simulink model "AOO_state"  (R2020a)
settings: Solver=FixedStepAuto  StartTime=0.0  StopTime=10.0  FixedStep=1e-3  RelTol=1e-3  EnableMultiTasking=on
undefined symbols (not defined in the file or in its folder): A1, D0, D1, D2, PTB3, PTB9, PTC16, PTC17
libraries: frdmk64flib x4
settings Model: ExtModeTrigDuration=5  Creator=John Sarga  LastModifiedBy=John Sarga
settings OptimizationCC: EnhancedBackFolding=on  PassReuseOutputArgsAs=Individual arguments  ZeroExternalMemoryAtStartup=off  ZeroInternalMemoryAtStartup=off  MaxStackSize=64  OptimizeBlockOrder=speed  DifferentSizesBufferReuse=on  OptimizationCustomize=off  EfficientTunableParamExpr=on
settings DebuggingCC: ParameterTunabilityLossMsg=error
settings HardwareCC: ProdBitPerPointer=32  ProdBitPerSizeT=32  ProdBitPerPtrDiffT=32  ProdLargestAtomicInteger=Long  ProdLargestAtomicFloat=Double  ProdWordSize=32  ProdHWDeviceType=ARM Compatible->ARM Cortex
settings SFSimCC: MATLABDynamicMemAlloc=off
settings RTWCC: SystemTargetFile=ert.tlc  HardwareBoard=NXP FRDM-K64F  TemplateMakefile=ert_default_tmf  Toolchain=GNU Tools for ARM Embedded Processors
settings CodeAppCC: ForceParamTrailComments=on  IgnoreCustomStorageClasses=off  OperatorAnnotations=on  SimulinkDataObjDesc=on  SFDataObjDesc=on  InsertBlockDesc=on

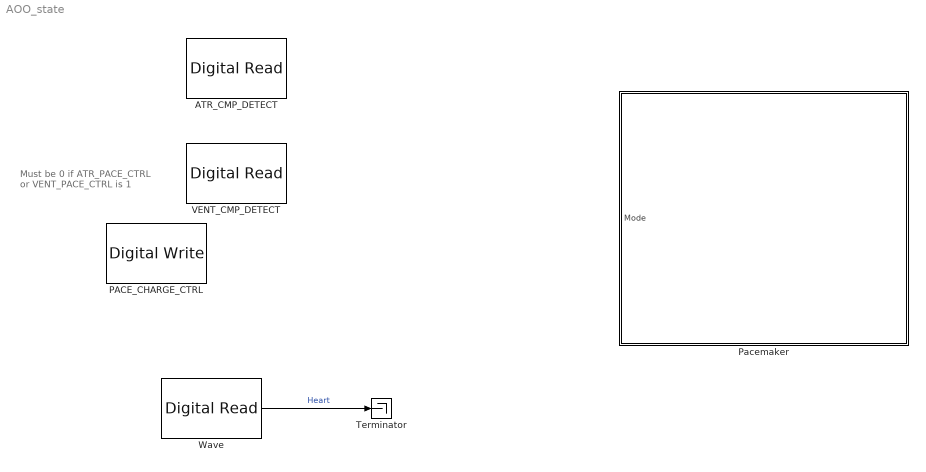
== system AOO_state ==
  note: Must be 0 if ATR_PACE_CTRL or VENT_PACE_CTRL
      | is 1
  ATR_CMP_DETECT : frdmk64flib/Digital Read  Whichpin=PTC16 (D0)  SampleTime=-1
  PACE_CHARGE_CTRL : frdmk64flib/Digital Write  Whichpin=PTB9 (D2)
  Pacemaker : Stateflow chart  TreatAsAtomicUnit=on
  Terminator : Terminator
  VENT_CMP_DETECT : frdmk64flib/Digital Read  Whichpin=PTC17 (D1)  SampleTime=-1
  Wave : frdmk64flib/Digital Read  Whichpin=PTB3 (A1)  SampleTime=-1
  wires:
  Wave/1 -> Terminator/1  "Heart"

== stateflow chart AOO_state/Pacemaker ==
  state Off
    Mode = Off
  state AOO
  (default) -> Off
  AOO -> Off : [Mode == Off]
  Off -> AOO : [Mode == AOO]
  data: Mode input Enum: PacemakerMode
